simulink model "HexC_FeedbackLinearizationController"  (R2022b)
settings: Solver=VariableStepAuto  StartTime=0.0  StopTime=tot_time  FixedStep=1e-2  RelTol=1e-3
InitFcn:
  | %% INITIALIZATION
  | 
  | A = [zeros(3, 3), eye(3); zeros(3, 6)];
  | 
  | B = [zeros(3, 3); eye(3)];
  | 
  | p = [-2 -2*10 -2*11 -2*12 -2*13 -2*14];
  | 
  | Kv = place(A, B, p);
  | 
  | Kp = Kv(:, 1:3);
  | Kd = Kv(:, 4:6);
  | 
  | p = [-20 -20*10 -20*11 -20*12 -20*13 -20*14];
  | 
  | Ke = place(A, B, p);
  | 
  | sigma = 10;
  | vi = 10;
  | D0 = eye(3)*10;
  | K0 = sigma*D0;
  | 
  | %% UAV PARAMETERS
  | 
  | mass = 2.4;
  | Ib = 2*diag([1.2416 1.2416 2*1.2416]);
  | 
  | %% ESTIMATOR PARAMETERS
  | 
  | syms s;
  | c_0 = 100;
  | poly = (s + c_0)^3;
  | K_est = double(coeffs(poly));
  | 
  | %% PLANNER (ASSUMING THE POINTS IN path HAVE ALREADY BEEN GENERATED WITH RRT)
  | Ts = 1e-3;
  | npoints = length(path(:, 1));
  | tseg = 5;
  | ttot=(npoints-1)*tseg; %duration
  | tdead=10; %dead time to evaluate the steady-state
  | tot_time = ttot + tdead;
  | 
  | t1=linspace(0,tseg,round(tseg/Ts));
  | t=linspace(0,ttot+tdead,round(ttot/Ts)+round(tdead/Ts));
  | 
  | phi_0 = deg2rad(0);
  | theta_0 = deg2rad(0);
  | psi_0 = deg2rad(0);
  | 
  | %p_d= zeros(4,length(t)); dot_p_d= zeros(4,length(t)); ddot_p_d= zeros(4,length(t));
  | p_d = []; dot_p_d = []; ddot_p_d = [];
  | 
  | for i = 1:npoints-1
  |     pi= zeros(6,length(t1)); dot_pi= zeros(6,length(t1)); ddot_pi= zeros(6,length(t1));
  |     %Initial and final conditions
  |     x0= path(i, 1); xf=path(i+1, 1); dot_x0= 0; dot_xf=0; ddot_x0=0; ddot_xf=0; dddot_x0 = 0; dddot_xf = 0;
  |     y0= path(i, 2); yf=path(i+1, 2); dot_y0= 0; dot_yf=0; ddot_y0=0; ddot_yf=0; dddot_y0 = 0; dddot_yf = 0;
  |     z0= path(i, 3); zf=path(i+1, 3); dot_z0= 0; dot_zf=0; ddot_z0=0; ddot_zf=0; dddot_z0 = 0; dddot_zf = 0;
  |     phi0 = phi_0+deg2rad(5*(i-1));
  |     phif=phi_0+deg2rad(5*i); dot_phi0= 0; dot_phif=0; ddot_phi0=0; ddot_phif=0; dddot_phi0 = 0; dddot_phif = 0;
  |     theta0 = theta_0+deg2rad(5*(i-1));
  |     thetaf=theta_0+deg2rad(5*i); dot_theta0= 0; dot_thetaf=0; ddot_theta0=0; ddot_thetaf=0; dddot_theta0 = 0; dddot_thetaf = 0;
  |     psi0 = psi_0+deg2rad(5*(i-1));
  |     psif=psi_0+deg2rad(5*i); dot_psi0= 0; dot_psif=0; ddot_psi0=0; ddot_psif=0; dddot_psi0 = 0; dddot_psif = 0;
  |     p0=[x0,y0,z0,phi0,theta0,psi0]; dot_p0=[dot_x0,dot_y0,dot_z0,dot_phi0,dot_theta0,dot_psi0]; ddot_p0=[ddot_x0,ddot_y0,ddot_z0,ddot_phi0,ddot_theta0,ddot_psi0]; dddot_p0=[dddot_x0,dddot_y0,dddot_z0,dddot_phi0,dddot_theta0,dddot_psi0];
  |     pf=[xf,yf,zf,phif,thetaf,psif]; dot_pf=[dot_xf,dot_yf,dot_zf,dot_phif,dot_thetaf,dot_psif]; ddot_pf=[ddot_xf,ddot_yf,ddot_zf,ddot_phif,ddot_thetaf,ddot_psif]; dddot_pf=[dddot_xf,dddot_yf,dddot_zf,dddot_phif,dddot_thetaf,dddot_psif];
  |     %5-th order polynomial
  |     a0=zeros(1,4); a1=zeros(1,4); a2=zeros(1,4); a3=zeros(1,4); a4=zeros(1,4); a5=zeros(1,4); a6 = zeros(1,4); a7 = zeros(1,4);
  | 
  |     t_iniz = 0;
  |     t_fin = tseg;
  | 
  |     for j=1:6
  |         A = [t_iniz^7, t_iniz^6, t_iniz^5, t_iniz^4, t_iniz^3, t_iniz^2, t_iniz, 1;
  |             t_fin^7, t_fin^6, t_fin^5, t_fin^4, t_fin^3, t_fin^2, t_fin, 1;
  |             7*t_iniz^6, 6*t_iniz^5, 5*t_iniz^4, 4*t_iniz^3, 3*t_iniz^2, 2*t_iniz, 1, 0;
  |             7*t_fin^6, 6*t_fin^5, 5*t_fin^4, 4*t_fin^3, 3*t_fin^2, 2*t_fin, 1, 0;
  |             42*t_iniz^5, 30*t_iniz^4, 20*t_iniz^3, 12*t_iniz^2, 6*t_iniz, 2, 0, 0;
  |             42*t_fin^5, 30*t_fin^4, 20*t_fin^3, 12*t_fin^2, 6*t_fin, 2, 0, 0;
  |             210*t_iniz^4, 120*t_iniz^3, 60*t_iniz^2, 24*t_iniz, 6, 0, 0, 0;
  |             210*t_fin^4, 120*t_fin^3, 60*t_fin^2, 24*t_fin, 6, 0, 0, 0];
  |         b = [p0(j) pf(j) dot_p0(j) dot_pf(j) ddot_p0(j) ddot_pf(j) dddot_p0(j) dddot_pf(j)]';
  |         a_temp = A\b;
  |         a7(j) = a_temp(1);
  |         a6(j) = a_temp(2);
  |         a5(j) = a_temp(3);
  |         a4(j) = a_temp(4);
  |         a3(j) = a_temp(5);
  |         a2(j) = a_temp(6);
  |         a1(j) = a_temp(7);
  |         a0(j) = a_temp(8);
  | 
  |         %trajectories
  |         pi(j,:)=a7(j)*t1.^7 + a6(j)*t1.^6 + a5(j)*t1.^5 +a4(j)*t1.^4 +a3(j)*t1.^3 +a2(j)*t1.^2 +a1(j)*(t1-(i-1)*tseg) +a0(j);
  |         dot_pi(j,:) = 7*a7(j)*t1.^6 + 6*a6(j)*t1.^5 + 5*a5(j)*t1.^4 +4*a4(j)*t1.^3 +3*a3(j)*t1.^2 +2*a2(j)*(t1-(i-1)*tseg) +a1(j);
  |         ddot_pi(j,:) = 42*a7(j)*t1.^5 + 30*a6(j)*t1.^4 + 5*4*a5(j)*t1.^3 +4*3*a4(j)*t1.^2 +3*2*a3(j)*(t1-(i-1)*tseg) +2*a2(j);
  |     end
  | 
  |     % figure(i)
  |     % plot(t1, pi)
  | 
  |     p_d = [p_d pi];
  |     dot_p_d = [dot_p_d dot_pi];
  |     ddot_p_d = [ddot_p_d ddot_pi];
  | 
  | end
  | 
  | %addition of the stead-state terms
  | p_d=[p_d zeros(1,round(tdead/Ts))+p_d(:, end)];
  | dot_p_d=[dot_p_d zeros(1,round(tdead/Ts))+dot_p_d(:, end)];
  | ddot_p_d=[ddot_p_d zeros(1,round(tdead/Ts))+ddot_p_d(:, end)];
  | %data for Simulink
  | pos_0 = [x0 y0 z0];
  | lin_vel_0 = [dot_x0 dot_y0 dot_z0];
  | w_bb_0 = [0 0 0];
  | csi_d=p_d(1:3,:); dot_csi_d=dot_p_d(1:3,:); ddot_csi_d=ddot_p_d(1:3,:);
  | phi_d=p_d(4,:); dot_phi_d=dot_p_d(4,:); ddot_phi_d=ddot_p_d(4,:);
  | theta_d=p_d(5,:); dot_theta_d=dot_p_d(5,:); ddot_theta_d=ddot_p_d(5,:);
  | psi_d=p_d(6,:); dot_psi_d=dot_p_d(6,:); ddot_psi_d=ddot_p_d(6,:);
values from neighbouring files (symbols this model uses):
  i = i+1    (= 1)    [PlannerRRT.m]
  j = j+0.5    (= 0.5)    [PlannerRRT.m]
  path = [path; roadmap(connections(indexPath-2, 2), :)]    [PlannerRRT.m]
undefined symbols (not defined in the file or in its folder): DiscIntNeverNeededParam
libraries: robotcorelib x1, uavutilslib x1
settings Model: Creator=Federico  LastModifiedBy=Federico

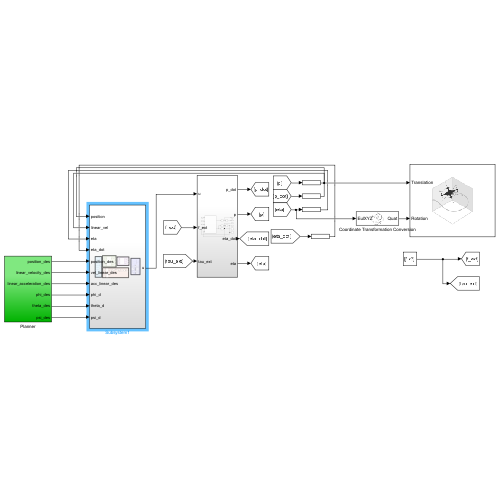
[thumbnail: Simulink's stored preview of the top-level diagram]
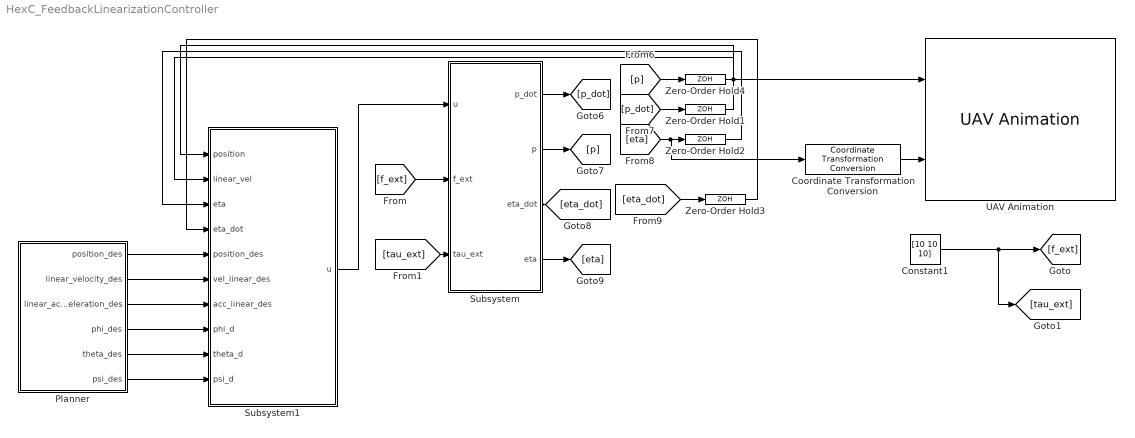
== system HexC_FeedbackLinearizationController ==
  Constant1 : Constant  Value=[10 10 10]
  Coordinate Transformation Conversion : robotcorelib/Coordinate Transformation Conversion  InputRepresentation=Euler Angles  InputEulerSequence=XYZ  ShowTrVecInputPort=on  OutputRepresentation=Quaternion  OutputEulerSequence=ZYX  ShowTrVecOutputPort=on  SimulateUsing=Interpreted execution
  Planner : Subsystem
  Subsystem : Subsystem
  Subsystem1 : Subsystem
  UAV Animation : uavutilslib/UAV Animation  UAVType=Multirotor  UAVSize=1  InertialZDirection=Down  SampleTime=0.01
  Zero-Order Hold{1..4} (4 alike) : ZeroOrderHold  SampleTime=Ts
  wires:
  Subsystem/4(eta) -> [eta]
  Subsystem/3(eta_dot) -> [eta_dot]
  [p] -> Zero-Order Hold4/1
  Subsystem/1(p_dot) -> [p_dot]
  [p_dot] -> Zero-Order Hold1/1
  Zero-Order Hold4/1 -> Subsystem1/1(position), UAV Animation/1
  Coordinate Transformation Conversion/1 -> UAV Animation/2
  [eta] -> Coordinate Transformation Conversion/1, Zero-Order Hold2/1
  Subsystem/2(p) -> [p]
  Zero-Order Hold1/1 -> Subsystem1/2(linear_vel)
  Zero-Order Hold2/1 -> Subsystem1/3(eta)
  [eta_dot] -> Zero-Order Hold3/1
  Zero-Order Hold3/1 -> Subsystem1/4(eta_dot)
  [f_ext] -> Subsystem/2(f_ext)
  [tau_ext] -> Subsystem/3(tau_ext)
  Subsystem1/1(u) -> Subsystem/1(u)
  Constant1/1 -> [tau_ext], [f_ext]
  Planner/4(phi_des) -> Subsystem1/8(phi_d)
  Planner/5(theta_des) -> Subsystem1/9(theta_d)
  Planner/1(position_des) -> Subsystem1/5(position_des)
  Planner/2(linear_velocity_des) -> Subsystem1/6(vel_linear_des)
  Planner/6(psi_des) -> Subsystem1/10(psi_d)
  Planner/3(linear_acceleration_des) -> Subsystem1/7(acc_linear_des)

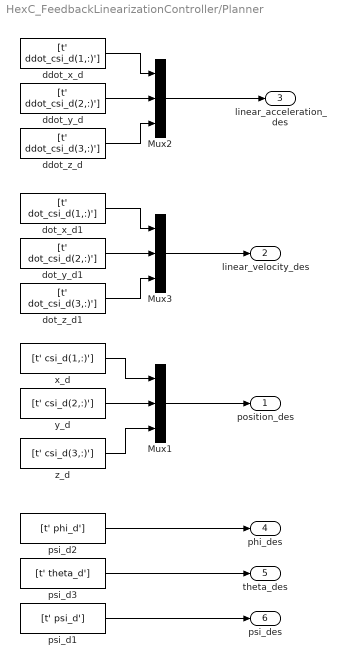
== system HexC_FeedbackLinearizationController/Planner ==
  Mux1 : Mux  Inputs=3
  Mux2 : Mux  Inputs=3
  Mux3 : Mux  Inputs=3
  ddot_x_d : FromWorkspace  VariableName=[t' ddot_csi_d(1,:)']  SampleTime=Ts
  ddot_y_d : FromWorkspace  VariableName=[t' ddot_csi_d(2,:)']  SampleTime=Ts
  ddot_z_d : FromWorkspace  VariableName=[t' ddot_csi_d(3,:)']  SampleTime=Ts
  dot_x_d1 : FromWorkspace  VariableName=[t' dot_csi_d(1,:)']  SampleTime=Ts
  dot_y_d1 : FromWorkspace  VariableName=[t' dot_csi_d(2,:)']  SampleTime=Ts
  dot_z_d1 : FromWorkspace  VariableName=[t' dot_csi_d(3,:)']  SampleTime=Ts
  psi_d1 : FromWorkspace  VariableName=[t' psi_d']  SampleTime=Ts
  psi_d2 : FromWorkspace  VariableName=[t' phi_d']  SampleTime=Ts
  psi_d3 : FromWorkspace  VariableName=[t' theta_d']  SampleTime=Ts
  x_d : FromWorkspace  VariableName=[t' csi_d(1,:)']  SampleTime=Ts
  y_d : FromWorkspace  VariableName=[t' csi_d(2,:)']  SampleTime=Ts
  z_d : FromWorkspace  VariableName=[t' csi_d(3,:)']  SampleTime=Ts
  position_des : Outport
  linear_velocity_des : Outport  Port=2
  linear_acceleration_des : Outport  Port=3
  phi_des : Outport  Port=4
  theta_des : Outport  Port=5
  psi_des : Outport  Port=6
  wires:
  y_d/1 -> Mux1/2
  z_d/1 -> Mux1/3
  x_d/1 -> Mux1/1
  ddot_y_d/1 -> Mux2/2
  ddot_z_d/1 -> Mux2/3
  ddot_x_d/1 -> Mux2/1
  Mux2/1 -> linear_acceleration_des/1
  Mux1/1 -> position_des/1
  dot_y_d1/1 -> Mux3/2
  dot_z_d1/1 -> Mux3/3
  dot_x_d1/1 -> Mux3/1
  Mux3/1 -> linear_velocity_des/1
  psi_d1/1 -> psi_des/1
  psi_d2/1 -> phi_des/1
  psi_d3/1 -> theta_des/1

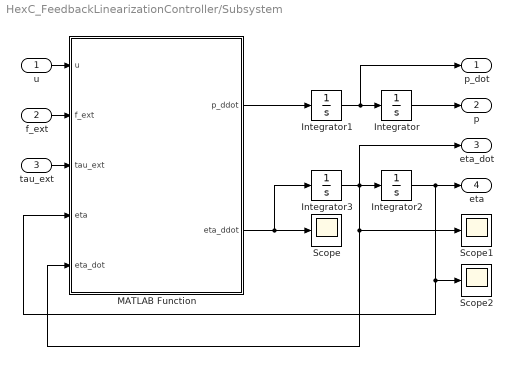
== system HexC_FeedbackLinearizationController/Subsystem ==
  u : Inport
  f_ext : Inport  Port=2
  tau_ext : Inport  Port=3
  Integrator : Integrator  InitialCondition=path(1, :)
  Integrator1 : Integrator
  Integrator2 : Integrator  InitialCondition=[0 0 psi_0]
  Integrator3 : Integrator
  MATLAB Function : MATLAB Function  TreatAsAtomicUnit=on
  Scope : Scope
  Scope1 : Scope
  Scope2 : Scope
  p_dot : Outport
  p : Outport  Port=2
  eta_dot : Outport  Port=3
  eta : Outport  Port=4
  wires:
  MATLAB Function/1(p_ddot) -> Integrator1/1
  Integrator1/1 -> p_dot/1, Integrator/1
  Integrator/1 -> p/1
  u/1 -> MATLAB Function/1(u)
  Integrator3/1 -> MATLAB Function/5(eta_dot), Scope1/1, eta_dot/1, Integrator2/1
  Integrator2/1 -> MATLAB Function/4(eta), Scope2/1, eta/1
  MATLAB Function/2(eta_ddot) -> Scope/1, Integrator3/1
  f_ext/1 -> MATLAB Function/2(f_ext)
  tau_ext/1 -> MATLAB Function/3(tau_ext)

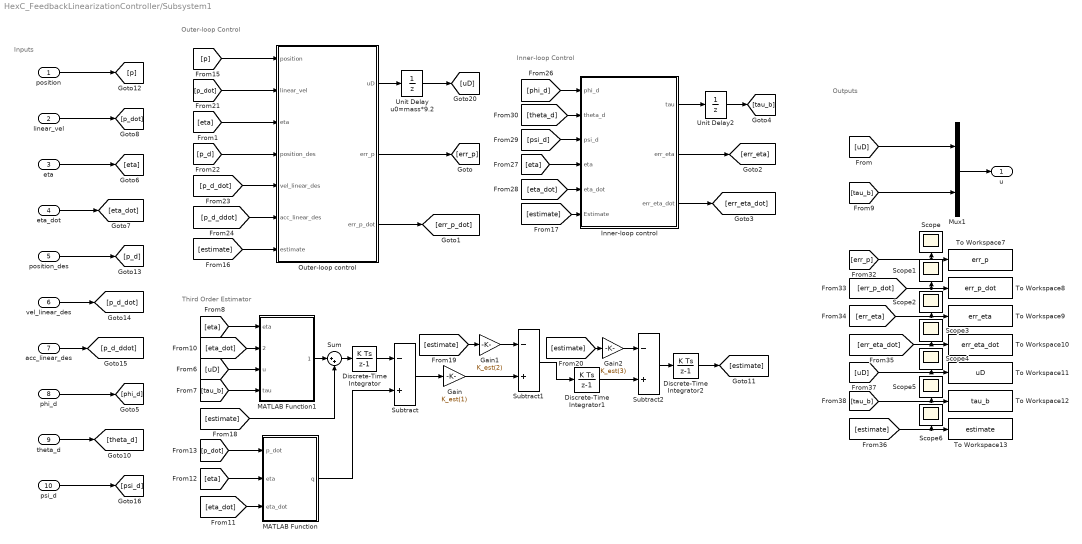
== system HexC_FeedbackLinearizationController/Subsystem1 ==
  note: Outer-loop Control
  note: Inner-loop Control
  note: Third Order Estimator
  note: Outputs
  note: Inputs
  position : Inport
  linear_vel : Inport  Port=2
  eta : Inport  Port=3
  eta_dot : Inport  Port=4
  position_des : Inport  Port=5
  vel_linear_des : Inport  Port=6
  acc_linear_des : Inport  Port=7
  phi_d : Inport  Port=8
  theta_d : Inport  Port=9
  psi_d : Inport  Port=10
  Discrete-Time Integrator : DiscreteIntegrator  SampleTime=-1  ICPrevOutput=DiscIntNeverNeededParam  ICPrevScaledInput=DiscIntNeverNeededParam
  Discrete-Time Integrator1 : DiscreteIntegrator  SampleTime=-1  ICPrevOutput=DiscIntNeverNeededParam  ICPrevScaledInput=DiscIntNeverNeededParam
  Discrete-Time Integrator2 : DiscreteIntegrator  SampleTime=-1  ICPrevOutput=DiscIntNeverNeededParam  ICPrevScaledInput=DiscIntNeverNeededParam
  Gain : Gain  Gain=K_est(1)
  Gain1 : Gain  Gain=K_est(2)
  Gain2 : Gain  Gain=K_est(3)
  Inner-loop control : Subsystem
  MATLAB Function : MATLAB Function  TreatAsAtomicUnit=on
  MATLAB Function1 : MATLAB Function  TreatAsAtomicUnit=on
  Mux1 : Mux  Inputs=2
  Outer-loop control : MATLAB Function  TreatAsAtomicUnit=on
  Scope{,1..6} (7 alike) : Scope
  Subtract : Sum  Inputs=-+
  Subtract1 : Sum  Inputs=-+
  Subtract2 : Sum  Inputs=-+
  Sum : Sum  Inputs=|++
  To Workspace10 : ToWorkspace  VariableName=err_eta_dot  SampleTime=-1
  To Workspace11 : ToWorkspace  VariableName=uD  SampleTime=-1
  To Workspace12 : ToWorkspace  VariableName=tau_b  SampleTime=-1
  To Workspace13 : ToWorkspace  VariableName=estimate  SampleTime=-1
  To Workspace7 : ToWorkspace  VariableName=err_p  SampleTime=-1
  To Workspace8 : ToWorkspace  VariableName=err_p_dot  SampleTime=-1
  To Workspace9 : ToWorkspace  VariableName=err_eta  SampleTime=-1
  Unit Delay u0=mass*9.2 : UnitDelay  InitialCondition=[0;0;mass*9.81]  SampleTime=Ts
  Unit Delay2 : UnitDelay  InitialCondition=[0 0 0]  SampleTime=Ts
  u : Outport
  wires:
  [p] -> Outer-loop control/1(position)
  [p_d] -> Outer-loop control/4(position_des)
  [p_dot] -> Outer-loop control/2(linear_vel)
  [p_d_dot] -> Outer-loop control/5(vel_linear_des)
  [p_d_ddot] -> Outer-loop control/6(acc_linear_des)
  [estimate] -> Outer-loop control/7(estimate)
  Unit Delay u0=mass*9.2/1 -> [uD]
  Outer-loop control/2(err_p) -> [err_p]
  Outer-loop control/3(err_p_dot) -> [err_p_dot]
  Outer-loop control/1(uD) -> Unit Delay u0=mass*9.2/1
  [theta_d] -> Inner-loop control/2(theta_d)
  [phi_d] -> Inner-loop control/1(phi_d)
  [eta] -> Inner-loop control/4(eta)
  [estimate] -> Inner-loop control/6(Estimate)
  [eta_dot] -> Inner-loop control/5(eta_dot)
  [psi_d] -> Inner-loop control/3(psi_d)
  Unit Delay2/1 -> [tau_b]
  Inner-loop control/2(err_eta) -> [err_eta]
  Inner-loop control/1(tau) -> Unit Delay2/1
  Inner-loop control/3(err_eta_dot) -> [err_eta_dot]
  [eta] -> MATLAB Function/2(eta)
  [estimate] -> Sum/2
  Gain2/1 -> Subtract2/1
  Subtract1/1 -> Discrete-Time Integrator1/1
  [eta_dot] -> MATLAB Function/3(eta_dot)
  Gain/1 -> Subtract1/2
  [p_dot] -> MATLAB Function/1(p_dot)
  [eta_dot] -> MATLAB Function1/2(eta_dot)
  [uD] -> MATLAB Function1/3(u)
  MATLAB Function1/1(model_term) -> Sum/1
  Discrete-Time Integrator/1 -> Subtract/1
  Sum/1 -> Discrete-Time Integrator/1
  MATLAB Function/1(q) -> Subtract/2
  [eta] -> MATLAB Function1/1(eta)
  [tau_b] -> MATLAB Function1/4(tau)
  Subtract2/1 -> Discrete-Time Integrator2/1
  Discrete-Time Integrator1/1 -> Subtract2/2
  Gain1/1 -> Subtract1/1
  [estimate] -> Gain2/1
  Subtract/1 -> Gain/1
  [estimate] -> Gain1/1
  Discrete-Time Integrator2/1 -> [estimate]
  [err_eta_dot] -> Scope3/1, To Workspace10/1
  [err_p] -> Scope/1, To Workspace7/1
  [tau_b] -> Mux1/2
  [err_eta] -> Scope2/1, To Workspace9/1
  [estimate] -> Scope6/1, To Workspace13/1
  [tau_b] -> Scope5/1, To Workspace12/1
  [err_p_dot] -> To Workspace8/1, Scope1/1
  Mux1/1 -> u/1
  [uD] -> Scope4/1, To Workspace11/1
  [eta] -> Outer-loop control/3(eta)
  eta/1 -> [eta]
  eta_dot/1 -> [eta_dot]
  position_des/1 -> [p_d]
  vel_linear_des/1 -> [p_d_dot]
  phi_d/1 -> [phi_d]
  position/1 -> [p]
  linear_vel/1 -> [p_dot]
  acc_linear_des/1 -> [p_d_ddot]
  psi_d/1 -> [psi_d]
  theta_d/1 -> [theta_d]
  [uD] -> Mux1/1

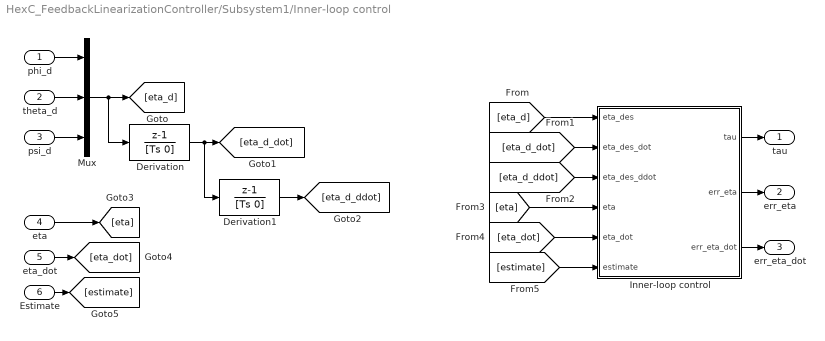
== system HexC_FeedbackLinearizationController/Subsystem1/Inner-loop control ==
  phi_d : Inport
  theta_d : Inport  Port=2
  psi_d : Inport  Port=3
  eta : Inport  Port=4
  eta_dot : Inport  Port=5
  Estimate : Inport  Port=6
  Derivation : DiscreteTransferFcn  Numerator=[1 -1]  Denominator=[Ts 0]  SampleTime=Ts
  Derivation1 : DiscreteTransferFcn  Numerator=[1 -1]  Denominator=[Ts 0]  SampleTime=Ts
  Inner-loop control : MATLAB Function  TreatAsAtomicUnit=on
  Mux : Mux  Inputs=3
  tau : Outport
  err_eta : Outport  Port=2
  err_eta_dot : Outport  Port=3
  wires:
  Inner-loop control/1(tau) -> tau/1
  phi_d/1 -> Mux/1
  theta_d/1 -> Mux/2
  psi_d/1 -> Mux/3
  Mux/1 -> [eta_d], Derivation/1
  Derivation/1 -> [eta_d_dot], Derivation1/1
  Derivation1/1 -> [eta_d_ddot]
  eta/1 -> [eta]
  eta_dot/1 -> [eta_dot]
  Estimate/1 -> [estimate]
  Inner-loop control/3(err_eta_dot) -> err_eta_dot/1
  Inner-loop control/2(err_eta) -> err_eta/1
  [eta_d] -> Inner-loop control/1(eta_des)
  [eta_d_dot] -> Inner-loop control/2(eta_des_dot)
  [eta_d_ddot] -> Inner-loop control/3(eta_des_ddot)
  [eta] -> Inner-loop control/4(eta)
  [eta_dot] -> Inner-loop control/5(eta_dot)
  [estimate] -> Inner-loop control/6(estimate)

== matlab function HexC_FeedbackLinearizationController/Subsystem1/MATLAB Function ==
  data: p_dot input size=3; q output size=6; eta input size=3; eta_dot input size=3; mass parameter size=1; Ib parameter size=[3,3]
function q = fcn(p_dot, eta, eta_dot, mass, Ib)

    phi = eta(1);
    theta = eta(2);
    psi = eta(3);
    phi_dot = eta_dot(1);
    theta_dot = eta_dot(2);
    psi_dot = eta_dot(3);
    Q = [1 0         -sin(theta);
         0 cos(phi)  cos(theta)*sin(phi);
         0 -sin(phi) cos(theta)*cos(phi)];
    Q_dot = [0 0                 -theta_dot*cos(theta);
             0 -phi_dot*sin(phi) -theta_dot*sin(theta)*sin(phi)+phi_dot*cos(theta)*cos(phi);
             0 -phi_dot*cos(phi) -theta_dot*sin(theta)*cos(phi)-phi_dot*cos(theta)*sin(phi)];
    M = Q'*Ib*Q;
    C = Q'*skew(Q*eta_dot)*Ib*Q+Q'*Ib*Q_dot;
    
    q = [mass*eye(3) zeros(3, 3);
         zeros(3, 3) M]*[p_dot; eta_dot];
    
end

function S = skew(v)
    if(numel(v)~= 1)
        S= [0 -v(3) v(2); 
            v(3) 0 -v(1);
            -v(2) v(1) 0];
    else
        S= zeros(3);
    end
end

== matlab function HexC_FeedbackLinearizationController/Subsystem/MATLAB Function ==
  data: u input size=6; f_ext input; tau_ext input; eta input size=3; eta_dot input size=3; mass parameter size=1; p_ddot output size=3; eta_ddot output size=3; Ib parameter size=[3, 3]

% UAV model
function [p_ddot, eta_ddot] = fcn(u, f_ext, tau_ext, eta, eta_dot, mass, Ib)

    g = 9.81;

    R = eul2rotm(eta', "XYZ");
    
    f = u(1:3);
   % f = R\u(1:3);
    tau = u(4:6); 

    phi = eta(1);
    theta = eta(2);
    psi = eta(3);
    phi_dot = eta_dot(1);
    theta_dot = eta_dot(2);
    psi_dot = eta_dot(3);
    Q = [1 0         -sin(theta);
         0 cos(phi)  cos(theta)*sin(phi);
         0 -sin(phi) cos(theta)*cos(phi)];
    Q_dot = [0 0                 -theta_dot*cos(theta);
             0 -phi_dot*sin(phi) -theta_dot*sin(theta)*sin(phi)+phi_dot*cos(theta)*cos(phi);
             0 -phi_dot*cos(phi) -theta_dot*sin(theta)*cos(phi)-phi_dot*cos(theta)*sin(phi)];
    M = Q'*Ib*Q;
    C = Q'*skew(Q*eta_dot)*Ib*Q+Q'*Ib*Q_dot;


    p_ddot = g*[0;0;1]-1/mass*R*f + f_ext/mass;
    eta_ddot = M\(-C*eta_dot+Q'*tau + tau_ext);

end

function S = skew(v)
    if(numel(v)~= 1)
        S= [0 -v(3) v(2); 
            v(3) 0 -v(1);
            -v(2) v(1) 0];
    else
        S= zeros(3);
    end
end

== matlab function HexC_FeedbackLinearizationController/Subsystem1/Outer-loop control ==
  data: uD output size=3; position input size=3; linear_vel input size=3; eta input size=3; mass parameter size=1; position_des input size=3; vel_linear_des input size=3; acc_linear_des input size=3; Kd parameter size=[3,3]; err_p output size=3; err_p_dot output size=3; estimate input size=6; Kp parameter size=[3,3]
function [uD, err_p, err_p_dot] = fcn(position, linear_vel, eta, mass, position_des, vel_linear_des, acc_linear_des, Kd, estimate, ...
Kp)

%% WRITE HERE THE OUTER-LOOP CONTROL

g = 9.81;

err_p = position - position_des;
err_p_dot = linear_vel - vel_linear_des;

R = eul2rotm(eta', 'XYZ');

uD = inv(R)*mass*([0;0;g]+1/mass*estimate(1:3)+Kp*err_p+Kd*err_p_dot-acc_linear_des);

== matlab function HexC_FeedbackLinearizationController/Subsystem1/Inner-loop control/Inner-loop control ==
  data: tau output size=3; eta_des input size=3; eta_des_dot input size=3; eta_des_ddot input size=3; eta input; eta_dot input; Ib parameter; estimate input size=6; sigma parameter size=1; vi parameter size=1; D0 parameter size=[3,3]; err_eta output; err_eta_dot output; K0 parameter size=[3,3]
function [tau, err_eta, err_eta_dot]  = fcn(eta_des, eta_des_dot, eta_des_ddot, eta, eta_dot, Ib, estimate, sigma, vi, D0, K0)

phi = eta(1);
theta = eta(2);
psi = eta(3);
phi_dot = eta_dot(1);
theta_dot = eta_dot(2);
psi_dot = eta_dot(3);
Q = [1 0         -sin(theta);
     0 cos(phi)  cos(theta)*sin(phi);
     0 -sin(phi) cos(theta)*cos(phi)];
Q_dot = [0 0                 -theta_dot*cos(theta);
         0 -phi_dot*sin(phi) -theta_dot*sin(theta)*sin(phi)+phi_dot*cos(theta)*cos(phi);
         0 -phi_dot*cos(phi) -theta_dot*sin(theta)*cos(phi)-phi_dot*cos(theta)*sin(phi)];
M = Q'*Ib*Q;
C = Q'*skew(Q*eta_dot)*Ib*Q+Q'*Ib*Q_dot;

err_eta = eta-eta_des;
err_eta_dot = eta_dot-eta_des_dot;
upsilon_eta = err_eta_dot+sigma*err_eta;
eta_r_dot = eta_des_dot-sigma*err_eta;
eta_r_ddot = eta_des_ddot-vi*err_eta_dot;

tau = Q'\(M*eta_r_ddot+C*eta_r_dot-estimate(4:6)-D0*upsilon_eta-K0*err_eta);

end

function S = skew(v)
    if(numel(v)~= 1)
        S= [0 -v(3) v(2); 
            v(3) 0 -v(1);
            -v(2) v(1) 0];
    else
        S= zeros(3);
    end
end

== matlab function HexC_FeedbackLinearizationController/Subsystem1/MATLAB Function1 ==
  data: eta input size=3; eta_dot input size=3; u input size=3; tau input size=3; model_term output size=6; mass parameter size=1; Ib parameter size=[3,3]
function model_term = fcn(eta, eta_dot, u, tau, mass, Ib)

    R = eul2rotm(eta', "XYZ");
    g = 9.81;
    
    phi = eta(1);
    theta = eta(2);
    psi = eta(3);
    phi_dot = eta_dot(1);
    theta_dot = eta_dot(2);
    psi_dot = eta_dot(3);
    Q = [1 0         -sin(theta);
         0 cos(phi)  cos(theta)*sin(phi);
         0 -sin(phi) cos(theta)*cos(phi)];
    Q_dot = [0 0                 -theta_dot*cos(theta);
             0 -phi_dot*sin(phi) -theta_dot*sin(theta)*sin(phi)+phi_dot*cos(theta)*cos(phi);
             0 -phi_dot*cos(phi) -theta_dot*sin(theta)*cos(phi)-phi_dot*cos(theta)*sin(phi)];
    M = Q'*Ib*Q;
    C = Q'*skew(Q*eta_dot)*Ib*Q+Q'*Ib*Q_dot;
    
    model_term = [mass*[0;0;g]-R*u;
        C'*eta_dot+Q'*tau];

end

function S = skew(v)
    if(numel(v)~= 1)
        S= [0 -v(3) v(2); 
            v(3) 0 -v(1);
            -v(2) v(1) 0];
    else
        S= zeros(3);
    end
end
